simulink model "LQR_slrt_2015a"  (R2015a)
settings: Solver=ode4  StartTime=0.0  StopTime=30  FixedStep=Ts  RelTol=1e-3
values from neighbouring files (symbols this model uses):
  dac_max = [3  ,17 , 0.5 , 0.2 , 0.2 ,1.5]    [initParams.m]    (also in teste.m)
  dac_min = [-7 ,5  ,-1.5 ,-0.4 ,-0.4 ,-3]    [initParams.m]    (also in teste.m)
libraries: slrtlib x2, xpcutilitieslib x1, xpcrtudplib x1, xpcmeasurementcomputinglib x1
settings Model: CovSFcnEnable=off  Creator=HIL  LastModifiedBy=zoero
settings SolverCC: EnableConcurrentExecution=on
settings DataIOCC: LimitDataPoints=off  MaxDataPoints=1e8
settings OptimizationCC: BlockReduction=off  OptimizeBlockIOStorage=off  BufferReuse=off  GlobalBufferReuse=off  ExpressionFolding=off  LocalBlockOutputs=off
settings DebuggingCC: SolverPrmCheckMsg=warning
settings HardwareCC: ProdIntDivRoundTo=Zero  ProdEndianess=LittleEndian  ProdLongLongMode=on  ProdHWDeviceType=Generic->32-bit x86 compatible
settings RTWCC: SystemTargetFile=slrt.tlc  TemplateMakefile=slrt_default_tmf  Description=Simulink Real-Time  RTWCompilerOptimization=on
settings SimulinkRealTimeCC: GeneratePreprocessorConditionals=Disable all  RL32LogTETModifier=off  RL32LogBufSizeModifier=10000000  xPCRL32EventNumber=100000

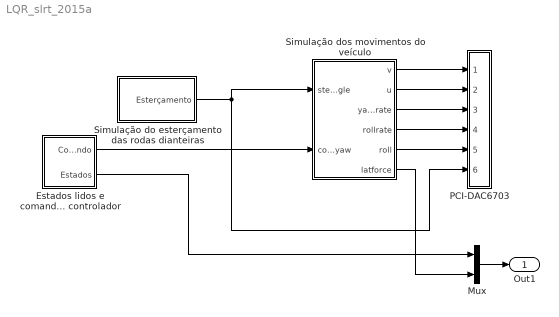
== system LQR_slrt_2015a ==
  Estados lidos e comando enviado pelo controlador : Subsystem
  Mux : Mux  Inputs=2
  PCI-DAC6703 : Subsystem
  "Simulação do esterçamento das rodas dianteiras " : Subsystem
  Simulação dos movimentos do veículo : Subsystem  TreatAsAtomicUnit=on
  Out1 : Outport
  wires:
  "Simulação do esterçamento das rodas dianteiras "/1(Esterçamento) -> Simulação dos movimentos do veículo/1(steer_angle), PCI-DAC6703/6(6)
  Estados lidos e comando enviado pelo controlador/1(Comando) -> Simulação dos movimentos do veículo/2(control_yaw)
  Simulação dos movimentos do veículo/1(v) -> PCI-DAC6703/1(1)
  Simulação dos movimentos do veículo/2(u) -> PCI-DAC6703/2(2)
  Simulação dos movimentos do veículo/3(yawrate) -> PCI-DAC6703/3(3)
  Simulação dos movimentos do veículo/4(rollrate) -> PCI-DAC6703/4(4)
  Simulação dos movimentos do veículo/5(roll) -> PCI-DAC6703/5(5)
  Estados lidos e comando enviado pelo controlador/2(Estados) -> Mux/1
  Simulação dos movimentos do veículo/6(latforce) -> Mux/2
  Mux/1 -> Out1/1

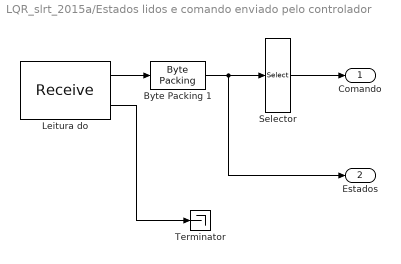
== system LQR_slrt_2015a/Estados lidos e comando enviado pelo controlador ==
  Byte Packing 1 : xpcutilitieslib/Byte Packing   MaskPackedDataType=double  MaskUnpackedDataTypes={'uint8'}  MaskAlignment=4
  "Leitura do " : xpcrtudplib/Legacy UDP/Receive   ipAddress=10.10.10.99  ipPort=65000  width=7*8  vblLen=off  sampletime=Ts
  Selector : Selector  InputPortWidth=7  Indices=[1]
  Terminator : Terminator
  Comando : Outport
  Estados : Outport  Port=2
  wires:
  "Leitura do "/1 -> Byte Packing 1/1
  "Leitura do "/2 -> Terminator/1
  Selector/1 -> Comando/1
  Byte Packing 1/1 -> Estados/1, Selector/1

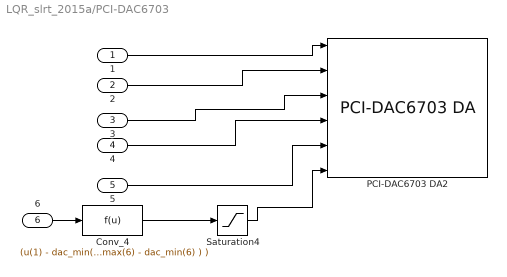
== system LQR_slrt_2015a/PCI-DAC6703 ==
  1 : Inport
  2 : Inport  Port=2
  3 : Inport  Port=3
  4 : Inport  Port=4
  5 : Inport  Port=5
  6 : Inport  Port=6
  Conv_4 : Fcn  Expr=(u(1) - dac_min(6))*(1.8/ (dac_max(6) - dac_min(6) ) )
  PCI-DAC6703 DA2 : xpcmeasurementcomputinglib/D//A/PCI-DAC6703 DA  channel=[1 2 3 4 5 6]  reset=[0 0 0 0 0 0]  initValue=[0 16.6667 0 0 0 0]  sampletime=Ts  slot=-1
  Saturation4 : Saturate  UpperLimit=1.8  LowerLimit=0
  wires:
  1/1 -> PCI-DAC6703 DA2/1
  2/1 -> PCI-DAC6703 DA2/2
  3/1 -> PCI-DAC6703 DA2/3
  4/1 -> PCI-DAC6703 DA2/4
  5/1 -> PCI-DAC6703 DA2/5
  Saturation4/1 -> PCI-DAC6703 DA2/6
  Conv_4/1 -> Saturation4/1
  6/1 -> Conv_4/1

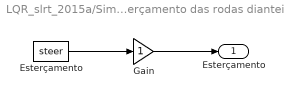
== system LQR_slrt_2015a/Simulação do esterçamento das rodas dianteiras  ==
  "Esterçamento " : FromWorkspace  VariableName=steer  SampleTime=0
  Gain : Gain
  Esterçamento : Outport
  wires:
  "Esterçamento "/1 -> Gain/1
  Gain/1 -> Esterçamento/1

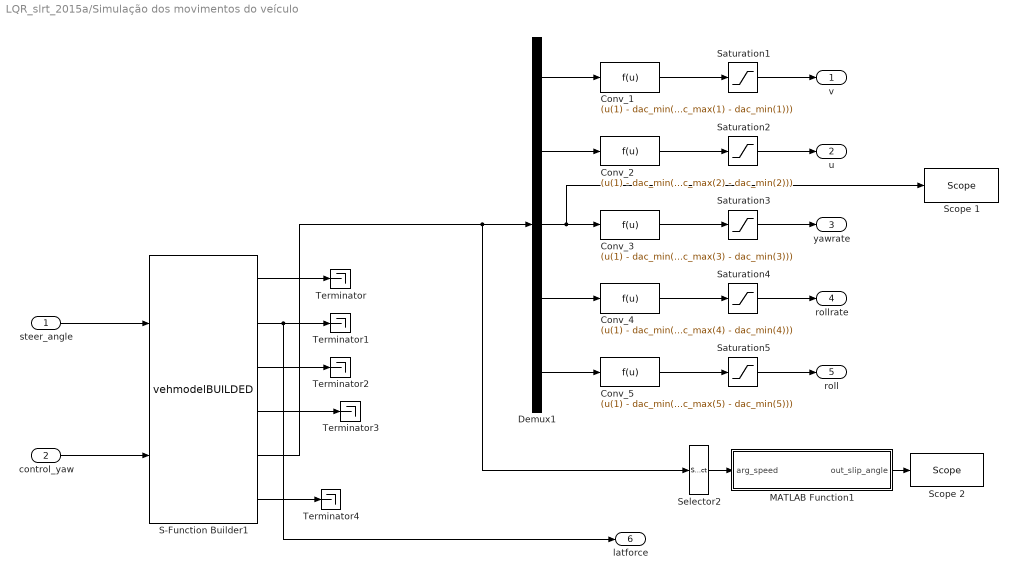
== system LQR_slrt_2015a/Simulação dos movimentos do veículo ==
  steer_angle : Inport
  control_yaw : Inport  Port=2
  Conv_1 : Fcn  Expr=(u(1) - dac_min(1))*(1.8/(dac_max(1) - dac_min(1)))
  Conv_2 : Fcn  Expr=(u(1) - dac_min(2))*(1.8/(dac_max(2) - dac_min(2)))
  Conv_3 : Fcn  Expr=(u(1) - dac_min(3))*(1.8/(dac_max(3) - dac_min(3)))
  Conv_4 : Fcn  Expr=(u(1) - dac_min(4))*(1.8/(dac_max(4) - dac_min(4)))
  Conv_5 : Fcn  Expr=(u(1) - dac_min(5))*(1.8/(dac_max(5) - dac_min(5)))
  Demux1 : Demux  Outputs=5
  MATLAB Function1 : MATLAB Function  TreatAsAtomicUnit=on
  S-Function Builder1 : S-Function  InitFcn=try, set_param(gcb,'FunctionName','vehmodelBUILDED'), end  FunctionName=vehmodelBUILDED  Parameters=params  SFunctionModules=vehmodelBUILDED_wrapper  mask(S-Function Builder){}
      mask help: Simulink:masks:SFunctionBuilder_MD
      mask init:
      | val = [[.9  0.75 0.75 1 1 .9 .9 1]',[1 1 0.75 0.75 .9 .9 1 .9]'];try , sys = get_param(gcb,'SfunBuilderFcnName');if isempty(sys), sys = get_param(gcb,'FunctionName'); end,catch, sys = get_param(gcb,'FunctionName'); end
      settings: CopyFcn=set_param(gcbh,'LinkStatus','none')  PreSaveFcn=try, set_param(gcb,'FunctionName','vehmodelBUILDED'), end  OpenFcn=sfunctionwizard(gcbh)
      mask Display: plot(val(:,1),val(:,2)),disp(sys), port_label('input',1,'inSteer'), port_label('input',2,'inMz'), port_label('output',1,'outFz'), port_label('output',2,'outFy'), port_label('output',3,'outFx'), port_label('output',4,'outSlip'), port_label('output',5,'outStates'), port_label('output',6,'outDStates')
  Saturation{1..5} (5 alike) : Saturate  UpperLimit=1.8  LowerLimit=0
  Scope 1 : slrtlib/Displays and Logging/Scope   scopeno=1  scopetype=Target  autostart=on  viewmode=Graphical sliding  formatstr='%15.6f'  grid=on  ylimits=[-pi,pi]  nosamples=5000  noprepostsamples=0  interleave=1  triggermode=FreeRun  triggersignal=1  trigsignalfromport=off  triggerlevel=0.0  triggerslope=Either  triggerscope=1  triggersample=0  filename=data.dat  mode=Lazy  writesize=512  autorestart=off  dynamicfilemode=off  maxwritefilesize=512*1024^2
  Scope 2 : slrtlib/Displays and Logging/Scope   scopeno=2  scopetype=Target  autostart=on  viewmode=Graphical sliding  formatstr='%15.6f'  grid=on  ylimits=[-20,20]  nosamples=5000  noprepostsamples=0  interleave=1  triggermode=FreeRun  triggersignal=1  trigsignalfromport=off  triggerlevel=0.0  triggerslope=Either  triggerscope=1  triggersample=0  filename=data.dat  mode=Lazy  writesize=512  autorestart=off  dynamicfilemode=off  maxwritefilesize=512*1024^2
  Selector2 : Selector  InputPortWidth=5  Indices=[1,2]
  Terminator{,1..4} (5 alike) : Terminator
  v : Outport
  u : Outport  Port=2
  yawrate : Outport  Port=3
  rollrate : Outport  Port=4
  roll : Outport  Port=5
  latforce : Outport  Port=6
  wires:
  control_yaw/1 -> S-Function Builder1/2
  steer_angle/1 -> S-Function Builder1/1
  S-Function Builder1/2 -> latforce/1, Terminator1/1
  S-Function Builder1/3 -> Terminator2/1
  S-Function Builder1/4 -> Terminator3/1
  Conv_1/1 -> Saturation1/1
  Conv_2/1 -> Saturation2/1
  Conv_3/1 -> Saturation3/1
  Conv_4/1 -> Saturation4/1
  Saturation3/1 -> yawrate/1
  Saturation4/1 -> rollrate/1
  Saturation2/1 -> u/1
  Saturation1/1 -> v/1
  Demux1/1 -> Conv_1/1
  Demux1/2 -> Conv_2/1
  Demux1/3 -> Scope 1/1, Conv_3/1
  Demux1/4 -> Conv_4/1
  S-Function Builder1/1 -> Terminator/1
  Conv_5/1 -> Saturation5/1
  Saturation5/1 -> roll/1
  Demux1/5 -> Conv_5/1
  S-Function Builder1/5 -> Selector2/1, Demux1/1
  Selector2/1 -> MATLAB Function1/1(arg_speed)
  MATLAB Function1/1(out_slip_angle) -> Scope 2/1
  S-Function Builder1/6 -> Terminator4/1

== matlab function LQR_slrt_2015a/Simulação dos movimentos do veículo/MATLAB Function1 ==
  data: arg_speed input; out_slip_angle output
function out_slip_angle = slipangle(arg_speed)

out_slip_angle = atan2(arg_speed(1),arg_speed(2));
